simulink subsystem "rss_PolarRefVltgCmpt"  (R2023a)
settings: Solver=VariableStepAuto  StartTime=0.0  StopTime=inf  RelTol=1e-3
undefined symbols (not defined in the file): Cdbl_uPhVltgMaxVal
libraries: lib_cart_to_polar_coor_transformer x1
settings Model: DefaultTestHarness=rss_PolarReferenceVoltageComputation_thu  Creator=RAN2OFO  LastModifiedBy=xiaoqiang.yuan
settings OptimizationCC: ReuseModelBlockBuffer=off

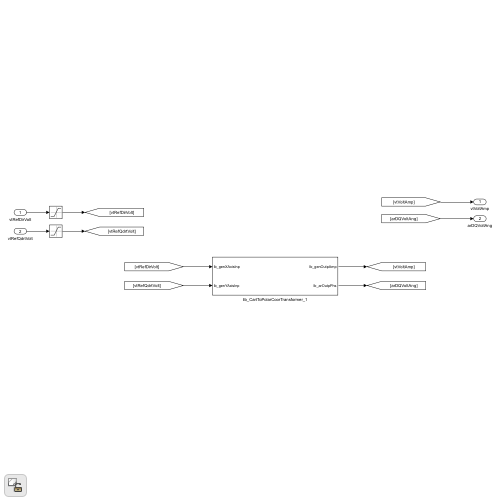
[thumbnail: Simulink's stored preview of the top-level diagram]
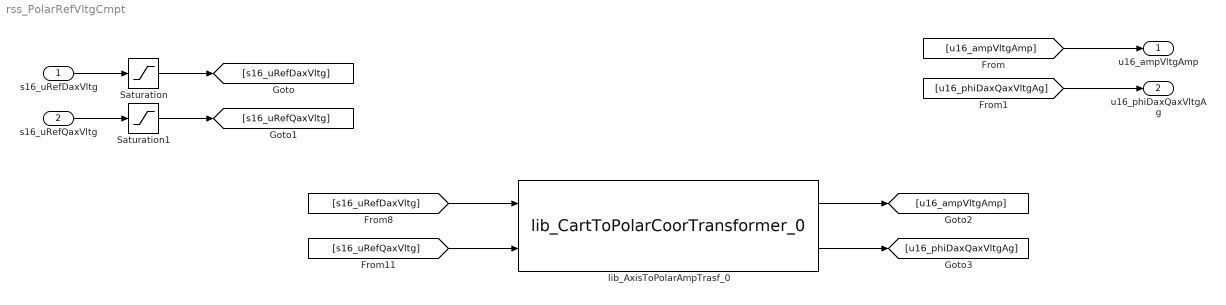
== system rss_PolarRefVltgCmpt ==
  s16_uRefDaxVltg : Inport  OutDataTypeStr=dt_Standardize_s16p15b0
  s16_uRefQaxVltg : Inport  Port=2  OutDataTypeStr=dt_Standardize_s16p15b0
  Saturation : Saturate  UpperLimit=Cdbl_uPhVltgMaxVal  LowerLimit=-Cdbl_uPhVltgMaxVal
  Saturation1 : Saturate  UpperLimit=Cdbl_uPhVltgMaxVal  LowerLimit=-Cdbl_uPhVltgMaxVal
  lib_AxisToPolarAmpTrasf_0 : lib_cart_to_polar_coor_transformer/lib_CartToPolarCoorTransformer_0  lb_parAsinLktSize=4095  lb_parAmpLktSize=512  lb_parOutpAmpDataType=dt_Standardize_u16p15b0
  u16_ampVltgAmp : Outport  OutDataTypeStr=dt_Standardize_u16p15b0
  u16_phiDaxQaxVltgAg : Outport  Port=2  OutDataTypeStr=dt_RadAng_u16r15b0
  wires:
  s16_uRefDaxVltg/1 -> Saturation/1
  s16_uRefQaxVltg/1 -> Saturation1/1
  [s16_uRefDaxVltg] -> lib_AxisToPolarAmpTrasf_0/1
  [s16_uRefQaxVltg] -> lib_AxisToPolarAmpTrasf_0/2
  Saturation/1 -> [s16_uRefDaxVltg]
  Saturation1/1 -> [s16_uRefQaxVltg]
  lib_AxisToPolarAmpTrasf_0/1 -> [u16_ampVltgAmp]
  [u16_ampVltgAmp] -> u16_ampVltgAmp/1
  [u16_phiDaxQaxVltgAg] -> u16_phiDaxQaxVltgAg/1
  lib_AxisToPolarAmpTrasf_0/2 -> [u16_phiDaxQaxVltgAg]
